simulink model "test10"  (R2024a)
settings: Solver=FixedStepAuto  StartTime=0.0  StopTime=30  FixedStep=0.001  MaxStep=1e-2  RelTol=1e-3
libraries: fl_lib x21, nesl_utility x14, simulink x7, sdl_lib x6
settings Model: DataDictionary=test4.sldd  Creator=18311  LastModifiedBy=18311

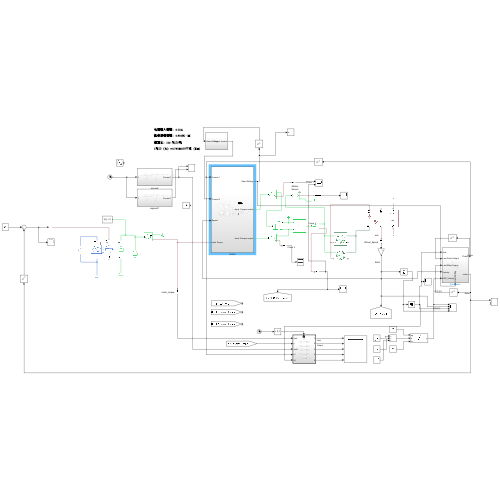
[thumbnail: Simulink's stored preview of the top-level diagram]
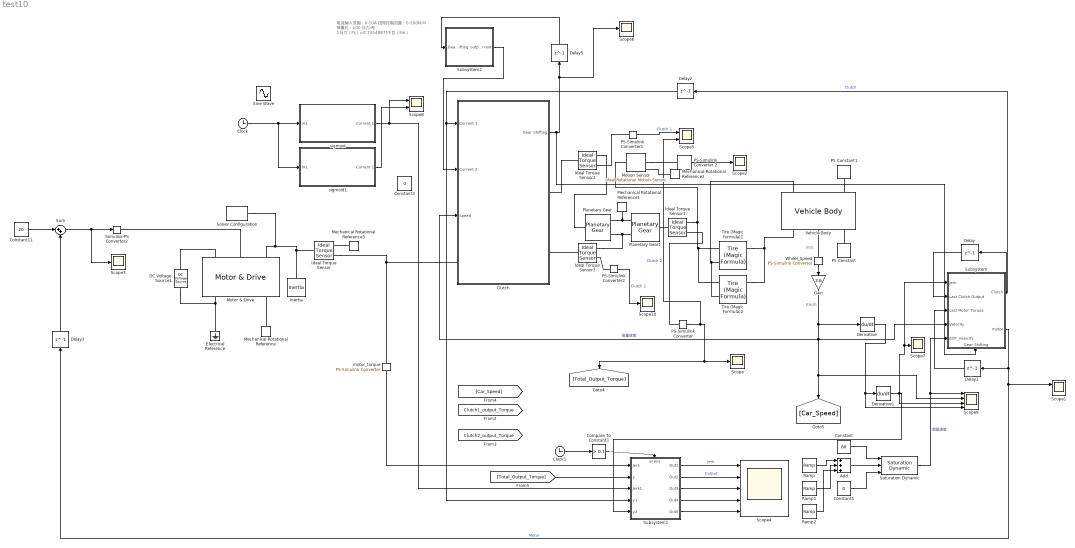
== system test10 ==
  note: Km/h
  note: m/s
  note: 电流输入范围：0-10A
      | 扭矩控制范围：0-500N·M
      | 推重比：100 马力/吨
      | 1马力（Ps）=0.73549875千瓦（Kw）
  Add : Sum  Inputs=+++
  Clock : Clock
  Clock1 : Clock
  Clutch : Subsystem
  Compare To Constant1 : simulink/Logic and Bit Operations/Compare To Constant  relop=>  const=0.1  OutDataTypeStr=boolean
  Constant : Constant  Value=80
  Constant1 : Constant  Value=0
  Constant11 : Constant  Value=20
  Constant3 : Constant  Value=0
  DC Voltage Source1 : fl_lib/Electrical/Electrical Sources/DC Voltage Source  v0=220 V
  Delay{,1..3,5} (5 alike) : Delay  DelayLength=1  InitialCondition=0
  Derivative : Derivative
  Derivative1 : Derivative
  Electrical Reference : fl_lib/Electrical/Electrical Elements/Electrical Reference
  Gain : Gain  Gain=3.6
  Ideal Torque Sensor{,1..3} (4 alike) : fl_lib/Mechanical/Mechanical Sensors/Ideal Torque Sensor
  Inertia : fl_lib/Mechanical/Rotational Elements/Inertia  inertia=0.01 kg*m^2  num_ports=foundation.enum.numPorts2.one  w_specify=off  w_priority=High  w=0 rad/s  w_nominal_specify=off  w_nominal_value=1  w_nominal_unit=rad/s  t_specify=off  t_priority=None  t=0 N*m  t_nominal_specify=off  t_nominal_value=1  t_nominal_unit=N*m
  Mechanical Rotational Reference{,1..3} (4 alike) : fl_lib/Mechanical/Rotational Elements/Mechanical Rotational Reference
  Motion Sensor : fl_lib/Mechanical/Mechanical Sensors/Ideal Rotational Motion Sensor  reference=foundation.enum.MeasurementReference.difference  acceleration_port=false  velocity_port=true  position_port=true  wrap_angle=simscape.enum.onoff.off  offset=0 rad
  Motor & Drive : sdl_lib/Engines & Motors/Motor & Drive  torque_max=200 N*m  power_max=73.549875 kW  Tc=0.02 s  eff=100  w_eff=4000 rpm  T_eff=200 N*m  thermal_port=simscape.enum.thermaleffects.omit  thermal_mass=100 J/K  temperature_specify=off  temperature_priority=High  temperature=300 K  temperature_nominal_specify=off  temperature_nominal_value=1  temperature_nominal_unit=K
      settings: InternalSimscapePortConfiguration="{\"Bottom\":[],\"Left\":[{\"id\":\"Vp\",\"label\":\"+\",\"type\":\"foundation.electrical.electrical\"},{\"id\":\"Tr\",\"label\":\"Tr\",\"type\":\"input\"},{\"id\":\"R\",\"label\":\"R\",\"type\":\"foundation.mechanical.rotational.rotational\"}],\"Right\":[{\"id\":\"Vm\",\"label\":\"-\",\"type\":\"foundation.electrical.electrical\"},{\"id\":\"Omega\",\"label\":\"w\",\"type\":\"output\"},{\"id\":\"C\",\"label\":\"C\",\"type\":\"foundation.mechanical.rotational.rotational\"}],\"Top\":[]}"
  PS Constant : fl_lib/Physical Signals/Sources/PS Constant  constant=0
  PS Constant1 : fl_lib/Physical Signals/Sources/PS Constant  constant=0
  PS-Simulink Converter : nesl_utility/PS-Simulink Converter  PhysicalDomain=network_engine_domain  SubClassName=ps_output  LeftPortType=input  RightPortType=output  PseudoPeriodic=off  Frequencies=[]  VectorFormat=inherit  Unit=inherit  AffineConversion=off
  PS-Simulink Converter 2 : nesl_utility/PS-Simulink Converter  PhysicalDomain=network_engine_domain  SubClassName=ps_output  LeftPortType=input  RightPortType=output  PseudoPeriodic=off  Frequencies=[]  VectorFormat=1-D array  Unit=rpm  AffineConversion=off
  PS-Simulink Converter1 : nesl_utility/PS-Simulink Converter  PhysicalDomain=network_engine_domain  SubClassName=ps_output  LeftPortType=input  RightPortType=output  PseudoPeriodic=off  Frequencies=[]  VectorFormat=inherit  Unit=inherit  AffineConversion=off
  PS-Simulink Converter2 : nesl_utility/PS-Simulink Converter  PhysicalDomain=network_engine_domain  SubClassName=ps_output  LeftPortType=input  RightPortType=output  PseudoPeriodic=off  Frequencies=[]  VectorFormat=inherit  Unit=inherit  AffineConversion=off
  Planetary Gear : sdl_lib/Gears/Planetary Gear  rs_ratio=1.5  friction_model=sdl.enum.gear_friction.none  efficiency=[.96, .98]  temperature_TLU=[280, 300, 320] K  efficiency_sp_TLU=[.95, .9, .85]  efficiency_rp_TLU=[.95, .9, .85]  pwr_thr=[.001, .001] W  mu_visc=[0, 0] N*m*s/rad  model_inertia=simscape.enum.onoff.off  planet_inertia=0.001 kg*m^2  thermal_mass=50 J/K  T_init=300 K
  Planetary Gear1 : sdl_lib/Gears/Planetary Gear  rs_ratio=3  friction_model=sdl.enum.gear_friction.none  efficiency=[.96, .98]  temperature_TLU=[280, 300, 320] K  efficiency_sp_TLU=[.95, .9, .85]  efficiency_rp_TLU=[.95, .9, .85]  pwr_thr=[.001, .001] W  mu_visc=[0, 0] N*m*s/rad  model_inertia=simscape.enum.onoff.off  planet_inertia=0.001 kg*m^2  thermal_mass=50 J/K  T_init=300 K
  Ramp : simulink/Sources/Ramp  slope=8  start=0  InitialOutput=0
  Ramp1 : simulink/Sources/Ramp  slope=-8  start=10  InitialOutput=0
  Ramp2 : simulink/Sources/Ramp  slope=-8  start=20  InitialOutput=0
  Saturation Dynamic : simulink/Discontinuities/Saturation Dynamic  OutMin=[]  OutMax=[]  OutDataTypeStr=Inherit: Same as second input  OutDataType=fixdt(1, 16)  OutScaling=2^-10  DoSatur=off
  Scope{,2..3,6..7,10} (6 alike) : Scope
  Scope1 : Scope  NumInputPorts=2
  Scope4 : Scope  NumInputPorts=5
  Scope5 : Scope  NumInputPorts=2
  Scope8 : Scope  NumInputPorts=2
  Scope9 : Scope  NumInputPorts=4
  Simulink-PS Converter2 : nesl_utility/Simulink-PS Converter  PhysicalDomain=network_engine_domain  SubClassName=ps_input  LeftPortType=input  RightPortType=output  PseudoPeriodic=off  Frequencies=[]  NoiseDistribution=none  NoiseParameters=[]  Unit=1  AffineConversion=off  FilteringAndDerivatives=provide  SimscapeFilterOrder=1  InputFilterTimeConstant=0.001  UdotUserProvided=0
  Sine Wave : Sin  Amplitude=5  Bias=5  SampleTime=0
  Solver Configuration : nesl_utility/Solver Configuration  PhysicalDomain=network_engine_domain  SubClassName=solver  LeftPortType=input  RightPortType=generic  Tones=[]  Harmonics=[]  SimulateNoise=off  Profile=off  UseLocalSampling=off  EnableSwitchedLinearOptims=on  FrequencyDomain=off  UseCCode=off  RelTol=0.001  AbsTol=0.001  MinStep=1e-09  ToWorkspace=off  RevertToSquareIcSolve=off  NumHomotopyIterations=100  PhasorMode=off  PhasorModeNumHarmonics=1  ConsistencySolver=NEWTON_XTOL_AFTER_FTOL  IndexReductionMethod=DerivativeReplacement  DoDC=off  ResidualTolerance=1e-09  ConsistencyTolSource=GLOBAL  ConsistencyAbsTol=0.001  ConsistencyRelTol=0.001  ConsistencyTolFactor=0.001  UseLocalSolver=off  LocalSolverChoice=NE_BACKWARD_EULER_ADVANCER  ResolveIndetEquations=on  FunctionEvalNumThread=1  LocalSolverSampleTime=0.001  DoFixedCost=off  MaxNonlinIter=3  MaxModeIter=2  ComputeImpulses=off  ImpulseIterations=2  LinearAlgebra=auto  LinearAlgebraNumThread=0  EquationFormulation=NE_TIME_EF  DelaysMemoryBudget=1024  AutomaticFiltering=on  FilteringTimeConstant=0.001  PartitionStorageMethod=AS_NEEDED  PartitionMemoryBudget=1024  PartitionMethod=ROBUST  MultibodyUseLocalSolver=off  MultibodyLocalSolverChoice=ODE1  MultibodyLocalSolverSampleTime=0.001
  Subsystem : Subsystem
      settings: PortSchema="{\"entries\":[{\"content\":{\"sides\":[{\"content\":{\"connectorIds\":[\"In1\",\"In2\",\"In3\",\"In4\",\"In5\"]},\"type\":\"ConnectorPlacement.EquallySpacedRectSide\",\"uuid\":\"5fc21831-6841-4d26-9c3b-273312b90933\"},{\"content\":{\"connectorIds\":[\"Out1\",\"Out2\"],\"side\":\"RIGHT\"},\"type\":\"ConnectorPlacement.EquallySpacedRectSide\",\"uuid\":\"d2976722-6716-4e73-9e66-a79e5a3f513c\"},{\"content\":{\"side\":\"TOP\"},\"type\":\"ConnectorPlacement.EquallySpacedRectSide\",\"uuid\":\"ab612606-baef-4711-bd49-fbf1df8d6358\"},{\"content\":{\"connectorIds\":[\"In6\"],\"side\":\"BOTTOM\"},\"type\":\"ConnectorPlacement.EquallySpacedRectSide\",\"uuid\":\"7be4a3f2-b973-419e-bcc3-9bfae442f3d1\"}]},\"type\":\"ConnectorPlacement.EquallySpacedConnector\",\"uuid\":\"4db5bfe9-dab6-4d88-a0f8-710cccb4717b\"}],\"packageUris\":[\"http://schema.mathworks.com/mf0/Connector/R2020b\"],\"version\":\"1.0\"}"
  Subsystem1 : Subsystem
  Subsystem2 : Subsystem
  Sum : Sum  Inputs=|++
  Tire (Magic Formula)1 : sdl_lib/Tires & Vehicles/Tire (Magic Formula)  parameterization=sdl.enum.magic_tire_model.peak  F_z1=2500 N  F_x1=3500 N  kappa1=10  B_m=10  C_m=1.9  D_m=1  E_m=0.97  fz0=4000 N  p_Cx=1.685  p_Dx=[1.21, -.037]  p_Ex=[.344, .095, -.02, 0]  p_Kx=[21.51, -.163, .245]  p_Hx=[-.002, .002]  p_Vx=[0, 0]  rolling_radius_model=sdl.enum.RollingRadiusParameterization.Constant  r_e=0.3 m  r_0=0.3 m  breff=8.39  dreff=0.26  freff=0.074  q_re0=0.99  q_v1=0.008  longvl=17 m/s  cz=5e5 N/m  model_resistance=true  resistance_model=sdl.enum.rollingResistanceParameterization.constant  coeff=0.015  p_tire=250e3 Pa  alpha=-0.003  beta=0.97  coeff_a=84e-4  coeff_b=6.2e-4 s/m  coeff_c=1.6e-4 s^2/m^2  p_tire0=240e3 Pa  fz0_resistance=4000 N  vH0=16 m/s  q_Sy=[.0082, 0, .0014, .001, 0, 0, 1.08, -.5]  v_thr=0.001 m/s  enable_scaling_coefficients=false  lfzO=1  lcx=1  lmux=1  lex=1  lkx=1  lhx=1  lvx=1  lmy=1  model_compliance=sdl.enum.compliance.off  stiffness=1e6 N/m  damping=1000 N*s/m  model_inertia=sdl.enum.model_inertia.off  inertia=1 kg*m^2  initial_velocity=0 rad/s  vxlow=1 m/s  v_tr_thr=0.1 m/s  kpumin=-1.5  kpumax=1.5
  Tire (Magic Formula)2 : sdl_lib/Tires & Vehicles/Tire (Magic Formula)  parameterization=sdl.enum.magic_tire_model.peak  F_z1=2500 N  F_x1=3000 N  kappa1=10  B_m=10  C_m=1.9  D_m=1  E_m=0.97  fz0=4000 N  p_Cx=1.685  p_Dx=[1.21, -.037]  p_Ex=[.344, .095, -.02, 0]  p_Kx=[21.51, -.163, .245]  p_Hx=[-.002, .002]  p_Vx=[0, 0]  rolling_radius_model=sdl.enum.RollingRadiusParameterization.Constant  r_e=0.3 m  r_0=0.3 m  breff=8.39  dreff=0.26  freff=0.074  q_re0=0.99  q_v1=0.008  longvl=17 m/s  cz=5e5 N/m  model_resistance=true  resistance_model=sdl.enum.rollingResistanceParameterization.constant  coeff=0.015  p_tire=250e3 Pa  alpha=-0.003  beta=0.97  coeff_a=84e-4  coeff_b=6.2e-4 s/m  coeff_c=1.6e-4 s^2/m^2  p_tire0=240e3 Pa  fz0_resistance=4000 N  vH0=16 m/s  q_Sy=[.0082, 0, .0014, .001, 0, 0, 1.08, -.5]  v_thr=0.001 m/s  enable_scaling_coefficients=false  lfzO=1  lcx=1  lmux=1  lex=1  lkx=1  lhx=1  lvx=1  lmy=1  model_compliance=sdl.enum.compliance.off  stiffness=1e6 N/m  damping=1000 N*s/m  model_inertia=sdl.enum.model_inertia.off  inertia=1 kg*m^2  initial_velocity=0 rad/s  vxlow=1 m/s  v_tr_thr=0.1 m/s  kpumin=-1.5  kpumax=1.5
  Vehicle Body : sdl_lib/Tires & Vehicles/Vehicle Body  mass=1000 kg  n_w=1  x_f=1.4 m  x_r=1.6 m  y_c=0.5 m  mass_var=simscape.enum.onoff.off  g=9.81 m/s^2  liftoff_warning=simscape.enum.onoff.off  area=3 m^2  Cd=0.4  rho=1.18 kg/m^3  model_pitch=simscape.enum.onoff.off  inertia=4000 kg*m^2  suspension_model=sdl.enum.linearTLU.linear  k_f=1e4 N/m  b_f=1e4 N*s/m  k_r=1e4 N/m  b_r=1e4 N*s/m  k_f_TLU=[-2000, -1000, 0, 1000, 2000] N  x_f_TLU=[-.4, -.2, 0, .2, .4] m  b_f_TLU=[-200, -100, 0, 100, 200] N  v_f_TLU=[-4, -2, 0, 2, 4] m/s  k_r_TLU=[-2000, -1000, 0, 1000, 2000] N  x_r_TLU=[-.4, -.2, 0, .2, .4] m  b_r_TLU=[-200, -100, 0, 100, 200] N  v_r_TLU=[-4, -2, 0, 2, 4] m/s  interp_method=simscape.enum.interpolation.linear  extrap_method=simscape.enum.extrapolation.linear  model_hardstop=simscape.enum.onoff.off  upper_bound_f=.25 m  lower_bound_f=-.25 m  stop_k_f=1e6 N/m  stop_b_f=150 N*s/m  upper_bound_r=.25 m  lower_bound_r=-.25 m  stop_k_r=1e6 N/m  stop_b_r=150 N*s/m  initial_pitch=0 rad  initial_pitch_rate=0 rad/s  v_specify=off  v_priority=High  v=0 m/s  v_nominal_specify=off  v_nominal_value=1  v_nominal_unit=m/s
  Wheel_Speed : nesl_utility/PS-Simulink Converter  PhysicalDomain=network_engine_domain  SubClassName=ps_output  LeftPortType=input  RightPortType=output  PseudoPeriodic=off  Frequencies=[]  VectorFormat=inherit  Unit=inherit  AffineConversion=off
  motor_torque : nesl_utility/PS-Simulink Converter  PhysicalDomain=network_engine_domain  SubClassName=ps_output  LeftPortType=input  RightPortType=output  PseudoPeriodic=off  Frequencies=[]  VectorFormat=inherit  Unit=inherit  AffineConversion=off
  sigmoid : Subsystem
  sigmoid1 : Subsystem
  wires:
  motor_torque/1 -> Subsystem1/1(Jerk)
  Wheel_Speed/1 -> Gain/1
  [Total_Output_Torque] -> Subsystem1/2(y)
  Derivative/1 -> Scope9/4, Derivative1/1
  Constant11/1 -> Sum/1
  Sum/1 -> Scope3/1, Simulink-PS Converter2/1
  Subsystem/2(motor) -> Delay3/1, Scope1/1, Delay1/1  "Motor"
  Subsystem/1(Clutch) -> Delay2/1, Delay/1  "Clutch"
  Derivative1/1 -> Scope7/1, Subsystem/1(Jerk), Scope9/3, Subsystem1/5(y2)
  sigmoid/1(Current 1) -> Scope8/1, Subsystem1/3(Jerk1)
  Clock/1 -> sigmoid1/1(In1), sigmoid/1(In1)
  Saturation Dynamic/1 -> Subsystem/5(EXP_Velocity), Scope9/1  "期望速度"
  Delay/1 -> Subsystem/2(Last Clutch Output)
  Delay1/1 -> Subsystem/3(Last Motor Torque)
  Delay2/1 -> Clutch/1(Current 1), Subsystem1/4(y1)
  Clock1/1 -> Compare To Constant1/1
  Compare To Constant1/1 -> Subsystem1/Enable
  Subsystem1/1(Out1) -> Scope4/1  "Jerk"
  Subsystem1/2(Out2) -> Scope4/2  "Output"
  Subsystem1/3(Out3) -> Scope4/3
  Subsystem1/4(Out4) -> Scope4/4
  Subsystem1/5(Out5) -> Scope4/5
  Constant/1 -> Saturation Dynamic/1
  Constant1/1 -> Saturation Dynamic/3
  Gain/1 -> Scope9/2, [Car_Speed], Clutch/3(Speed), Subsystem/4(Velocity), Derivative/1  "测量速度"
  sigmoid1/1(Current 1) -> Scope8/2
  Delay3/1 -> Sum/2
  PS-Simulink Converter/1 -> Scope5/2, [Total_Output_Torque], Scope/1  "Clutch 2"
  PS-Simulink Converter 2/1 -> Scope2/1
  PS-Simulink Converter1/1 -> Scope5/1  "Clutch 1"
  Clutch/1(Gear Shifting) -> Subsystem/6(Gear Shifting), Scope6/1, Delay5/1
  Delay5/1 -> Subsystem2/1(Gear shifting)
  Subsystem2/1(output current) -> Clutch/2(Current 2)
  PS-Simulink Converter2/1 -> Scope10/1  "Clutch 2"
  Ramp/1 -> Add/1
  Ramp1/1 -> Add/2
  Ramp2/1 -> Add/3
  Add/1 -> Saturation Dynamic/2
  connections:
  Motor & Drive/LConn1 -- DC Voltage Source1/LConn1
  Electrical Reference/LConn1 -- DC Voltage Source1/RConn1 -- Motor & Drive/RConn1
  Mechanical Rotational Reference/LConn1 -- Motor & Drive/RConn3
  Inertia/LConn1 -- Motor & Drive/LConn3 -- Solver Configuration/RConn1 -- Ideal Torque Sensor/LConn1
  PS Constant/RConn1 -- Vehicle Body/LConn3
  PS Constant1/RConn1 -- Vehicle Body/RConn3
  Ideal Torque Sensor/RConn2 -- motor_torque/LConn1 -- Clutch/LConn1
  Wheel_Speed/LConn1 -- Vehicle Body/LConn2
  Simulink-PS Converter2/RConn1 -- Motor & Drive/LConn2
  Tire (Magic Formula)1/RConn2 -- Tire (Magic Formula)2/RConn2 -- Vehicle Body/LConn1
  Tire (Magic Formula)1/LConn1 -- Tire (Magic Formula)2/LConn1 -- Vehicle Body/RConn1
  Mechanical Rotational Reference3/LConn1 -- Ideal Torque Sensor/RConn1
  Planetary Gear/RConn1 -- Mechanical Rotational Reference1/LConn1 -- Planetary Gear1/RConn1
  Ideal Torque Sensor1/LConn1 -- Planetary Gear1/LConn1
  PS-Simulink Converter/LConn1 -- Ideal Torque Sensor1/RConn2
  Planetary Gear/RConn2 -- Ideal Torque Sensor3/RConn1 -- Planetary Gear1/RConn2
  Motion Sensor/RConn2 -- PS-Simulink Converter 2/LConn1
  Ideal Torque Sensor1/RConn1 -- Tire (Magic Formula)2/LConn2 -- Tire (Magic Formula)1/LConn2 -- Motion Sensor/LConn1
  Mechanical Rotational Reference2/LConn1 -- Motion Sensor/RConn1
  Ideal Torque Sensor2/RConn1 -- Planetary Gear/LConn1
  PS-Simulink Converter1/LConn1 -- Ideal Torque Sensor2/RConn2
  Ideal Torque Sensor2/LConn1 -- Clutch/RConn1
  Ideal Torque Sensor3/LConn1 -- Clutch/RConn2
  PS-Simulink Converter2/LConn1 -- Ideal Torque Sensor3/RConn2

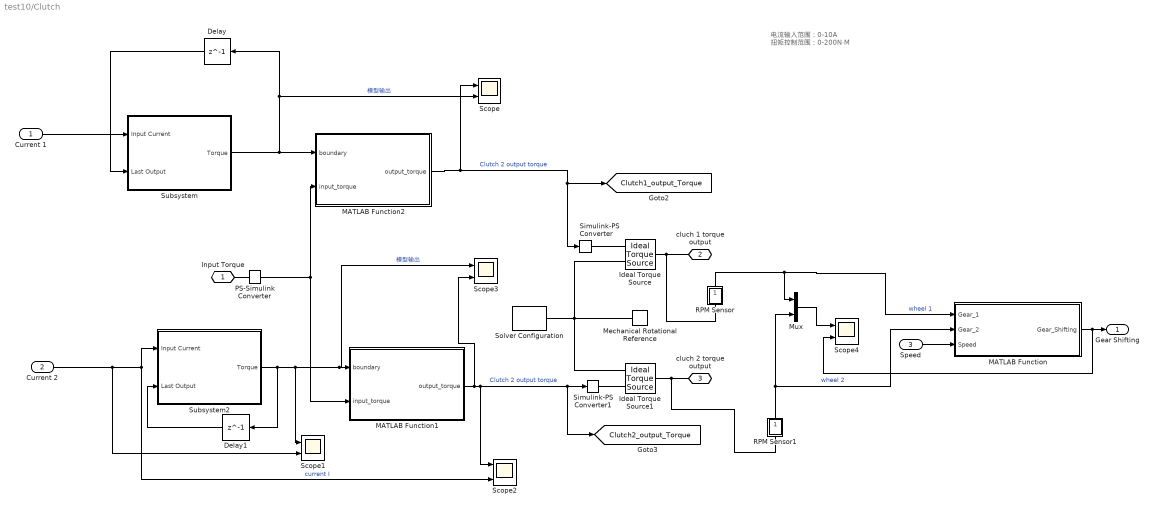
== system test10/Clutch ==
  note: 电流输入范围：0-10A
      | 扭矩控制范围：0-200N·M
  Current 1 : Inport
  Current 2 : Inport  Port=2
  Speed : Inport  Port=3
  Delay : Delay  DelayLength=1  InitialCondition=0
  Delay1 : Delay  DelayLength=1  InitialCondition=0
  Ideal Torque Source : fl_lib/Mechanical/Mechanical Sources/Ideal Torque Source
  Ideal Torque Source1 : fl_lib/Mechanical/Mechanical Sources/Ideal Torque Source
  MATLAB Function : MATLAB Function  TreatAsAtomicUnit=on
  MATLAB Function1 : MATLAB Function  TreatAsAtomicUnit=on
  MATLAB Function2 : MATLAB Function  TreatAsAtomicUnit=on
  Mechanical Rotational Reference : fl_lib/Mechanical/Rotational Elements/Mechanical Rotational Reference
  Mux : Mux  Inputs=2
  PS-Simulink Converter : nesl_utility/PS-Simulink Converter  PhysicalDomain=network_engine_domain  SubClassName=ps_output  LeftPortType=input  RightPortType=output  PseudoPeriodic=off  Frequencies=[]  VectorFormat=inherit  Unit=inherit  AffineConversion=off
  RPM Sensor : Subsystem
      mask Display: disp('S')
  RPM Sensor1 : Subsystem
      mask Display: disp('S')
  Scope{,1,3..4} (4 alike) : Scope  NumInputPorts=2
  Scope2 : Scope  NumInputPorts=3
  Simulink-PS Converter : nesl_utility/Simulink-PS Converter  PhysicalDomain=network_engine_domain  SubClassName=ps_input  LeftPortType=input  RightPortType=output  PseudoPeriodic=off  Frequencies=[]  NoiseDistribution=none  NoiseParameters=[]  Unit=1  AffineConversion=off  FilteringAndDerivatives=provide  SimscapeFilterOrder=1  InputFilterTimeConstant=0.001  UdotUserProvided=0
  Simulink-PS Converter1 : nesl_utility/Simulink-PS Converter  PhysicalDomain=network_engine_domain  SubClassName=ps_input  LeftPortType=input  RightPortType=output  PseudoPeriodic=off  Frequencies=[]  NoiseDistribution=none  NoiseParameters=[]  Unit=1  AffineConversion=off  FilteringAndDerivatives=provide  SimscapeFilterOrder=1  InputFilterTimeConstant=0.001  UdotUserProvided=0
  Solver Configuration : nesl_utility/Solver Configuration  PhysicalDomain=network_engine_domain  SubClassName=solver  LeftPortType=input  RightPortType=generic  Tones=[]  Harmonics=[]  SimulateNoise=off  Profile=off  UseLocalSampling=off  EnableSwitchedLinearOptims=on  FrequencyDomain=off  UseCCode=off  RelTol=0.001  AbsTol=0.001  MinStep=1e-09  ToWorkspace=off  RevertToSquareIcSolve=off  NumHomotopyIterations=100  PhasorMode=off  PhasorModeNumHarmonics=1  ConsistencySolver=NEWTON_XTOL_AFTER_FTOL  IndexReductionMethod=DerivativeReplacement  DoDC=off  ResidualTolerance=1e-09  ConsistencyTolSource=GLOBAL  ConsistencyAbsTol=0.001  ConsistencyRelTol=0.001  ConsistencyTolFactor=0.001  UseLocalSolver=off  LocalSolverChoice=NE_BACKWARD_EULER_ADVANCER  ResolveIndetEquations=on  FunctionEvalNumThread=1  LocalSolverSampleTime=0.001  DoFixedCost=off  MaxNonlinIter=3  MaxModeIter=2  ComputeImpulses=off  ImpulseIterations=2  LinearAlgebra=auto  LinearAlgebraNumThread=0  EquationFormulation=NE_TIME_EF  DelaysMemoryBudget=1024  AutomaticFiltering=on  FilteringTimeConstant=0.001  PartitionStorageMethod=AS_NEEDED  PartitionMemoryBudget=1024  PartitionMethod=ROBUST  MultibodyUseLocalSolver=off  MultibodyLocalSolverChoice=ODE1  MultibodyLocalSolverSampleTime=0.001
  Subsystem : Subsystem  mask{c=-2, k=20, d=0.6, alpha=-37.209}
  Subsystem2 : Subsystem  mask{c=-2, k=20, d=0.6, alpha=-37.209}
  Input Torque : PMIOPort  Side=Left
  cluch 1 torque output : PMIOPort  Port=2  Side=Right
  cluch 2 torque output : PMIOPort  Port=3  Side=Right
  Gear Shifting : Outport
  tag scope: Clutch1_output_Torque=global, Clutch2_output_Torque=global
  wires:
  Current 1/1 -> Subsystem/1(Input Current)
  Current 2/1 -> Scope1/2, Scope2/3, Subsystem2/1(Input Current)  "current I"
  MATLAB Function1/1(output_torque) -> Scope3/2, [Clutch2_output_Torque], Simulink-PS Converter1/1, Scope2/1  "Clutch 2 output torque"
  MATLAB Function2/1(output_torque) -> Scope/1, Simulink-PS Converter/1, [Clutch1_output_Torque]  "Clutch 2 output torque"
  PS-Simulink Converter/1 -> MATLAB Function2/2(input_torque), MATLAB Function1/2(input_torque)
  RPM Sensor/1(rpm) -> Mux/1, MATLAB Function/1(Gear_1)  "wheel 1"
  Subsystem2/1(Torque) -> Delay1/1, Scope1/1, Scope3/1, MATLAB Function1/1(boundary)  "模型输出"
  RPM Sensor1/1(rpm) -> Mux/2, MATLAB Function/2(Gear_2)  "wheel 2"
  Subsystem/1(Torque) -> Delay/1, Scope/2, MATLAB Function2/1(boundary)  "模型输出"
  Speed/1 -> MATLAB Function/3(Speed)
  MATLAB Function/1(Gear_Shifting) -> Scope4/2, Gear Shifting/1
  Mux/1 -> Scope4/1
  Delay/1 -> Subsystem/2(Last Output)
  Delay1/1 -> Subsystem2/2(Last Output)
  connections:
  Input Torque/RConn1 -- PS-Simulink Converter/LConn1
  Ideal Torque Source/RConn2 -- Ideal Torque Source1/RConn2 -- Mechanical Rotational Reference/LConn1 -- Solver Configuration/RConn1
  Ideal Torque Source/LConn1 -- RPM Sensor/LConn1 -- cluch 1 torque output/RConn1
  Ideal Torque Source1/LConn1 -- RPM Sensor1/LConn1 -- cluch 2 torque output/RConn1
  Ideal Torque Source/RConn1 -- Simulink-PS Converter/RConn1
  Ideal Torque Source1/RConn1 -- Simulink-PS Converter1/RConn1

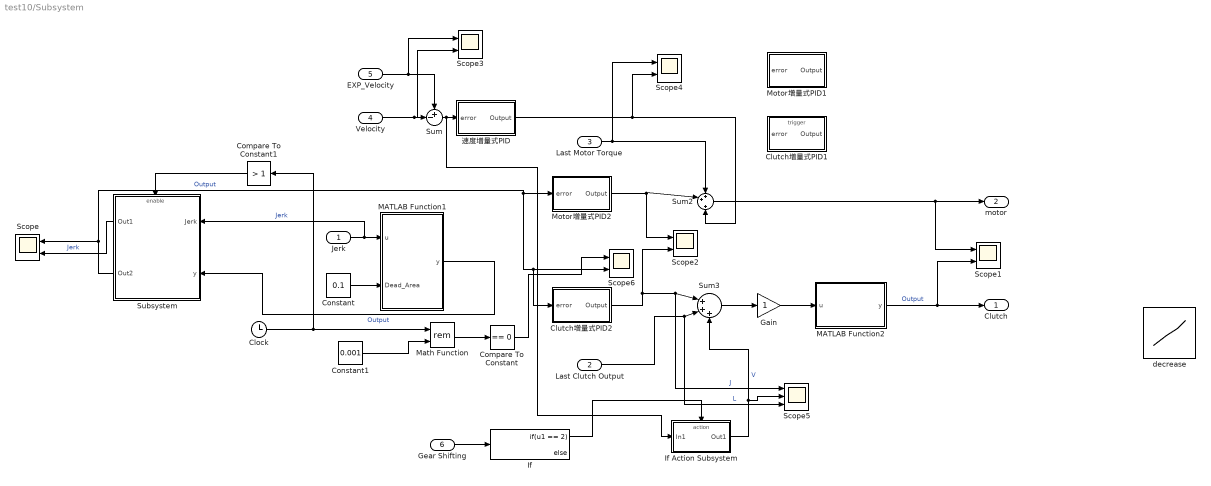
== system test10/Subsystem ==
  Jerk : Inport
  Last Clutch Output : Inport  Port=2
  Last Motor Torque : Inport  Port=3
  Velocity : Inport  Port=4
  EXP_Velocity : Inport  Port=5
  Gear Shifting : Inport  Port=6
  Clock : Clock
  Clutch增量式PID1 : Subsystem  mask{Kp=0.09, Ki=0.02, Kd=0.03}
      mask DialogControl ParameterGroupVar Prompt: 参数
  Clutch增量式PID2 : Subsystem  mask{Kp=0.0002, Ki=0, Kd=0.00001}
      mask DialogControl ParameterGroupVar Prompt: 参数
  Compare To Constant : simulink/Logic and Bit Operations/Compare To Constant  relop===  const=0  OutDataTypeStr=boolean
  Compare To Constant1 : simulink/Logic and Bit Operations/Compare To Constant  relop=>  const=1  OutDataTypeStr=boolean
  Constant : Constant  Value=0.1
  Constant1 : Constant  Value=0.001
  Gain : Gain
  If : If  IfExpression=u1 == 2
  If Action Subsystem : Subsystem  TreatAsAtomicUnit=on
  MATLAB Function1 : MATLAB Function  TreatAsAtomicUnit=on
  MATLAB Function2 : MATLAB Function  TreatAsAtomicUnit=on
  Math Function : Math  Operator=rem
  Motor增量式PID1 : Subsystem  mask{Kp=5, Ki=1, Kd=3}
      mask DialogControl ParameterGroupVar Prompt: 参数
  Motor增量式PID2 : Subsystem  mask{Kp=0, Ki=0, Kd=0}
      mask DialogControl ParameterGroupVar Prompt: 参数
  Scope{,1..4,6} (6 alike) : Scope  NumInputPorts=2
  Scope5 : Scope  NumInputPorts=3
  Subsystem : Subsystem
  Sum : Sum  Inputs=+-|
  Sum2 : Sum  Inputs=++|+
  Sum3 : Sum  Inputs=|+++
  decrease : Lookup_n-D  NumberOfTableDimensions=1  BreakpointsForDimension1=[5.5594823336345e-05;6.14417460221472e-05;6.79035869809514e-05;7.50450159711001e-05;8.29375037389161e-05;9.16600371985333e-05;0.000101299909808739;0.000111953595051133;0.000123727711744276;0.000136740090845997;0.000151120954409751;0.000167014218480952;0.00018457893295667;0.000203990872799214;0.000225444296504455;0.000249153889394299;0.000275356911145835;0.000304315569005653;0.000336319640386712;0.000371689371028895;0.000410778677647633;0.000453978687024344;0.000501721646837642;0.000554485247227949;0.000612797396166024;0.000677241496197702;0.000748462275106112;0.000827172228516664;0.000914158738521614;0.00101029193907773;0.00111653340629563;0.00123394575986232;0.00136370327079497;0.00150710358059758;0.00166558064777336;0.00184071904963424;0.00203426978055207;0.00224816770233296;0.00248455081839335;0.00274578156101333;0.00303447030028919;0.00335350130466478;0.00370606140626397;0.00409567164986051;0.00452622223240535;0.00500201107079564;0.00552778636923599;0.00610879359434402;0.00675082730632838;0.00746028833836698;0.00824424686398295;0.00911051194400646;0.0100677082008564;0.0111253603286032;0.0122939862127742;0.0135851995042896;0.0150118225673699;0.0165880108017442;0.0183293894249281;0.0202532038904988;0.0223784852127633;0.0247262315663477;0.0273196076301106;0.0301841632470842;0.0333480730741335;0.0368423989943599;0.0407013771589613;0.0449627316094118;0.0496680165005697;0.0548629889945041;0.0605980149158412;0.0669285092428486;0.0739154134428198;0.081625711531599;0.0901329865284782;0.0995180186690433;0.109869426305932;0.121284349842742;0.133869178276648;0.147740316932731;0.163024993714409;0.179862099620916;0.198403057340775;0.218812709361305;0.241270214176692;0.265969935768659;0.293122307513563;0.322954646984505;0.355711892726362;0.391657227967644;0.431072549410861;0.474258731775668;0.521535630784177;0.573241758988688;0.629733560569965;0.691384203433468;0.758581800212436;0.831726964939224;0.911229610148562;0.997504891196852;1.09096821195613;1.19202922022118;1.30108474362998;1.41851064900488;1.54465265083535;1.67981614866076;1.82425523806356;1.97816111441418;2.14165016957441;2.31475216500982;2.49739894404882;2.68941421369995;2.89050497374996;3.10025518872388;3.31812227831834;3.54343693774205;3.77540668798146;4.01312339887548;4.25557483188341;4.50166002687522;4.7502081252106;5;5.2497918747894;5.49833997312478;5.74442516811659;5.98687660112452;6.22459331201854;6.45656306225795;6.68187772168166;6.89974481127612;7.10949502625004;7.31058578630005;7.50260105595118;7.68524783499018;7.85834983042559;8.02183888558582;8.17574476193644;8.32018385133924;8.45534734916465;8.58148935099512;8.69891525637002;8.80797077977882;8.90903178804387;9.00249510880315;9.08877038985144;9.16827303506078;9.24141819978757;9.30861579656653;9.37026643943003;9.42675824101131;9.47846436921582;9.52574126822433;9.56892745058914;9.60834277203236;9.64428810727364;9.67704535301549;9.70687769248644;9.73403006423134;9.75872978582331;9.78118729063869;9.80159694265923;9.82013790037908;9.83697500628559;9.85225968306727;9.86613082172335;9.87871565015726;9.89013057369407;9.90048198133096;9.90986701347152;9.9183742884684;9.92608458655718;9.93940198508416;9.94513701100549;9.95503726839059;9.96665192692587;9.97527376843365;9.9949979889292;9.99993209641302]  Table=[0;6.14417460221472e-05;6.79035869809514e-05;7.50450159711001e-05;8.29375037389161e-05;9.16600371985333e-05;0.000101299909808739;0.000111953595051133;0.000123727711744276;0.000136740090845997;0.000151120954409752;0.000167014218480952;0.00018457893295667;0.000203990872799214;0.000225444296504455;0.000249153889394299;0.000275356911145835;0.000304315569005653;0.000336319640386712;0.000371689371028895;0.000410778677647633;0.000453978687024344;0.000501721646837643;0.000554485247227949;0.000612797396166024;0.000677241496197702;0.000748462275106112;0.000827172228516664;0.000914158738521614;0.00101029193907773;0.00111653340629563;0.00123394575986232;0.00136370327079497;0.00150710358059758;0.00166558064777336;0.00184071904963424;0.00203426978055207;0.00224816770233296;0.00248455081839335;0.00274578156101333;0.00303447030028919;0.00335350130466478;0.00370606140626397;0.00409567164986051;0.00452622223240536;0.00500201107079564;0.00552778636923599;0.00610879359434402;0.00675082730632838;0.00746028833836698;0.00824424686398295;0.00911051194400646;0.0100677082008564;0.0111253603286032;0.0122939862127742;0.0135851995042896;0.0150118225673699;0.0165880108017442;0.0183293894249281;0.0202532038904988;0.0223784852127634;0.0247262315663477;0.0273196076301106;0.0301841632470842;0.0333480730741335;0.0368423989943599;0.0407013771589613;0.0449627316094118;0.0496680165005697;0.0548629889945041;0.0605980149158412;0.0669285092428486;0.0739154134428198;0.081625711531599;0.0901329865284782;0.0995180186690433;0.109869426305932;0.121284349842742;0.133869178276648;0.147740316932731;0.163024993714409;0.179862099620916;0.198403057340775;0.218812709361305;0.241270214176692;0.265969935768659;0.293122307513563;0.322954646984505;0.355711892726362;0.391657227967644;0.431072549410861;0.474258731775668;0.521535630784177;0.573241758988688;0.629733560569965;0.691384203433468;0.758581800212436;0.831726964939224;0.911229610148562;0.997504891196852;1.09096821195613;1.19202922022118;1.30108474362998;1.41851064900488;1.54465265083535;1.67981614866076;1.82425523806356;1.97816111441418;2.14165016957441;2.31475216500982;2.49739894404882;2.68941421369995;2.89050497374996;3.10025518872388;3.31812227831834;3.54343693774205;3.77540668798146;4.01312339887548;4.25557483188341;4.50166002687522;4.7502081252106;5;5.2497918747894;5.49833997312478;5.74442516811659;5.98687660112452;6.22459331201854;6.45656306225795;6.68187772168166;6.89974481127612;7.10949502625004;7.31058578630005;7.50260105595118;7.68524783499018;7.85834983042559;8.02183888558582;8.17574476193644;8.32018385133924;8.45534734916465;8.58148935099512;8.69891525637002;8.80797077977882;8.90903178804387;9.00249510880315;9.08877038985144;9.16827303506078;9.24141819978757;9.30861579656653;9.37026643943003;9.42675824101131;9.47846436921582;9.52574126822433;9.56892745058914;9.60834277203236;9.64428810727364;9.67704535301549;9.70687769248644;9.73403006423134;9.75872978582331;9.78118729063869;9.80159694265923;9.82013790037908;9.83697500628559;9.85225968306727;9.86613082172335;9.87871565015726;9.89013057369407;9.90048198133096;9.90986701347152;9.9183742884684;9.92608458655718;9.93307149075715;9.93940198508416;9.94513701100549;9.95503726839059;9.96665192692587;9.97527376843365;9.98641480049571;]  InternalRulePriority=Speed  RndMeth=Simplest
  速度增量式PID : Subsystem  mask{Kp=20, Ki=0.2, Kd=0}
      mask DialogControl ParameterGroupVar Prompt: 参数
  Clutch : Outport
  motor : Outport  Port=2
  wires:
  Velocity/1 -> Scope3/2, Sum/2
  EXP_Velocity/1 -> Scope3/1, Sum/1
  Jerk/1 -> Subsystem/1(Jerk), MATLAB Function1/1(u)  "Jerk"
  速度增量式PID/1(Output) -> Scope4/2, Sum2/3
  Last Motor Torque/1 -> Sum2/1, Scope4/1
  Motor增量式PID2/1(Output) -> Scope2/1, Sum2/2
  Last Clutch Output/1 -> Scope5/3, Sum3/2  "L"
  Sum/1 -> If Action Subsystem/1(In1), 速度增量式PID/1(error)
  MATLAB Function1/1(y) -> Subsystem/2(y)  "Output"
  Constant/1 -> MATLAB Function1/2(Dead_Area)
  Sum2/1 -> Scope1/1, motor/1
  Sum3/1 -> Gain/1
  Clock/1 -> Compare To Constant1/1, Math Function/1
  Constant1/1 -> Math Function/2
  Math Function/1 -> Compare To Constant/1
  Compare To Constant/1 -> Scope6/1
  Gain/1 -> MATLAB Function2/1(u)
  MATLAB Function2/1(y) -> Scope1/2, Clutch/1  "Output"
  Compare To Constant1/1 -> Subsystem/Enable
  Subsystem/2(Out2) -> Scope/1, Clutch增量式PID2/1(error), Scope6/2, Motor增量式PID2/1(error)  "Output"
  Clutch增量式PID2/1(Output) -> Scope2/2, Scope5/1, Sum3/1  "J"
  Gear Shifting/1 -> If/1
  If/1 -> If Action Subsystem/Action
  If Action Subsystem/1(Out1) -> Scope5/2, Sum3/3  "V"
  Subsystem/1(Out1) -> Scope/2  "Jerk"

== system test10/Subsystem1 ==
  Jerk : Inport
  y : Inport  Port=2
  Jerk1 : Inport  Port=3
  y1 : Inport  Port=4
  y2 : Inport  Port=5
  Enable : EnablePort
  Out1 : Outport
  Out2 : Outport  Port=2
  Out3 : Outport  Port=3
  Out4 : Outport  Port=4
  Out5 : Outport  Port=5
  wires:
  Jerk/1 -> Out1/1
  y/1 -> Out2/1
  Jerk1/1 -> Out3/1
  y1/1 -> Out4/1
  y2/1 -> Out5/1

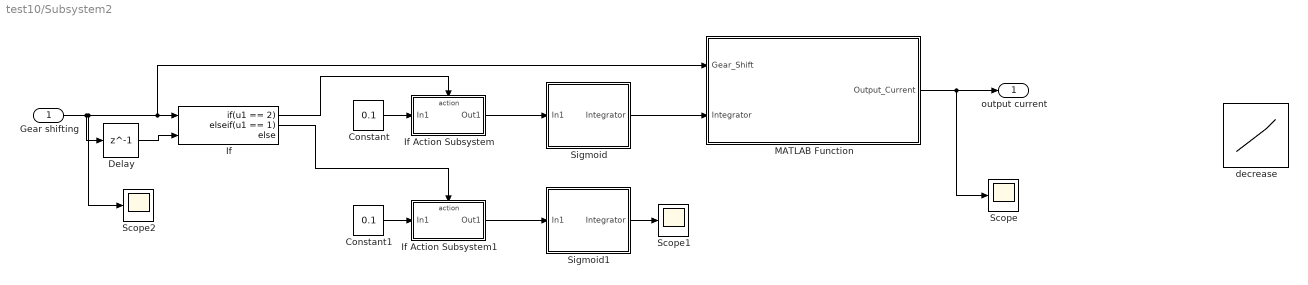
== system test10/Subsystem2 ==
  Gear shifting : Inport
  Constant : Constant  Value=0.1
  Constant1 : Constant  Value=0.1
  Delay : Delay  DelayLength=1  InitialCondition=0
  If : If  NumInputs=2  IfExpression=u1 == 2  ElseIfExpressions=u1 == 1
  If Action Subsystem : Subsystem  TreatAsAtomicUnit=on
  If Action Subsystem1 : Subsystem  TreatAsAtomicUnit=on
  MATLAB Function : MATLAB Function  TreatAsAtomicUnit=on
  Scope : Scope
  Scope1 : Scope
  Scope2 : Scope
  Sigmoid : Subsystem
  Sigmoid1 : Subsystem
  decrease : Lookup_n-D  NumberOfTableDimensions=1  BreakpointsForDimension1=[0:1:10]  Table=10*1./(1+exp(-[0:1:10]+5))  InternalRulePriority=Speed  RndMeth=Simplest
  output current : Outport
  wires:
  Gear shifting/1 -> Scope2/1, MATLAB Function/1(Gear_Shift), If/1, Delay/1
  If/1 -> If Action Subsystem/Action
  Constant/1 -> If Action Subsystem/1(In1)
  If Action Subsystem/1(Out1) -> Sigmoid/1(In1)
  MATLAB Function/1(Output_Current) -> Scope/1, output current/1
  Sigmoid/1(Integrator) -> MATLAB Function/2(Integrator)
  Constant1/1 -> If Action Subsystem1/1(In1)
  If Action Subsystem1/1(Out1) -> Sigmoid1/1(In1)
  Delay/1 -> If/2
  If/2 -> If Action Subsystem1/Action
  Sigmoid1/1(Integrator) -> Scope1/1

== system test10/sigmoid ==
  In1 : Inport
  Constant : Constant
  Constant1 : Constant  Value=-50
  Constant2 : Constant  Value=-1
  Gain : Gain  Gain=10
  Gain1 : Gain  Gain=5
  Math Function : Math  Operator=pow
  Math Function1 : Math
  Sum : Sum  Inputs=|++
  Sum1 : Sum  Inputs=|++
  Current 1 : Outport
  wires:
  Constant1/1 -> Sum/2
  In1/1 -> Gain1/1
  Sum/1 -> Math Function1/1
  Math Function1/1 -> Sum1/2
  Constant/1 -> Sum1/1
  Constant2/1 -> Math Function/2
  Sum1/1 -> Math Function/1
  Math Function/1 -> Gain/1
  Gain/1 -> Current 1/1
  Gain1/1 -> Sum/1

== system test10/sigmoid1 ==
  In1 : Inport
  Constant : Constant
  Constant1 : Constant  Value=50
  Constant2 : Constant  Value=-1
  Gain : Gain  Gain=10
  Gain1 : Gain  Gain=-5
  Math Function : Math  Operator=pow
  Math Function1 : Math
  Sum : Sum  Inputs=|++
  Sum1 : Sum  Inputs=|++
  Current 1 : Outport
  wires:
  Constant1/1 -> Sum/2
  In1/1 -> Gain1/1
  Sum/1 -> Math Function1/1
  Math Function1/1 -> Sum1/2
  Constant/1 -> Sum1/1
  Constant2/1 -> Math Function/2
  Sum1/1 -> Math Function/1
  Math Function/1 -> Gain/1
  Gain/1 -> Current 1/1
  Gain1/1 -> Sum/1

== system test10/Clutch/RPM Sensor ==
  Mechanical Rotational Reference : fl_lib/Mechanical/Rotational Elements/Mechanical Rotational Reference
  Motion Sensor : fl_lib/Mechanical/Mechanical Sensors/Ideal Rotational Motion Sensor  reference=foundation.enum.MeasurementReference.difference  acceleration_port=false  velocity_port=true  position_port=true  wrap_angle=simscape.enum.onoff.off  offset=0 rad
  PS-Simulink Converter 2 : nesl_utility/PS-Simulink Converter  PhysicalDomain=network_engine_domain  SubClassName=ps_output  LeftPortType=input  RightPortType=output  PseudoPeriodic=off  Frequencies=[]  VectorFormat=1-D array  Unit=rpm  AffineConversion=off
  R : PMIOPort  Side=Left
  rpm : Outport  VectorParamsAs1DForOutWhenUnconnected=off
  wires:
  PS-Simulink Converter 2/1 -> rpm/1
  connections:
  R/RConn1 -- Motion Sensor/LConn1
  Motion Sensor/RConn1 -- Mechanical Rotational Reference/LConn1
  Motion Sensor/RConn2 -- PS-Simulink Converter 2/LConn1

== system test10/Clutch/RPM Sensor1 ==
  Mechanical Rotational Reference : fl_lib/Mechanical/Rotational Elements/Mechanical Rotational Reference
  Motion Sensor : fl_lib/Mechanical/Mechanical Sensors/Ideal Rotational Motion Sensor  reference=foundation.enum.MeasurementReference.difference  acceleration_port=false  velocity_port=true  position_port=true  wrap_angle=simscape.enum.onoff.off  offset=0 rad
  PS-Simulink Converter 2 : nesl_utility/PS-Simulink Converter  PhysicalDomain=network_engine_domain  SubClassName=ps_output  LeftPortType=input  RightPortType=output  PseudoPeriodic=off  Frequencies=[]  VectorFormat=1-D array  Unit=rpm  AffineConversion=off
  R : PMIOPort  Side=Left
  rpm : Outport  VectorParamsAs1DForOutWhenUnconnected=off
  wires:
  PS-Simulink Converter 2/1 -> rpm/1
  connections:
  R/RConn1 -- Motion Sensor/LConn1
  Motion Sensor/RConn1 -- Mechanical Rotational Reference/LConn1
  Motion Sensor/RConn2 -- PS-Simulink Converter 2/LConn1

== system test10/Clutch/Subsystem ==
  Input Current : Inport
  Last Output : Inport  Port=2
  Abs : Abs  SaturateOnIntegerOverflow=off
  Derivative : Derivative
  If Action Subsystem : Subsystem  TreatAsAtomicUnit=on
  If Action Subsystem1 : Subsystem  TreatAsAtomicUnit=on
  If1 : If  IfExpression=u1 <= 200
  Merge : Merge
  Scope : Scope  NumInputPorts=3
  Torque : Outport
  wires:
  Input Current/1 -> Scope/1, If Action Subsystem1/1(Input Current), Derivative/1
  If1/1 -> If Action Subsystem1/Action
  If1/2 -> If Action Subsystem/Action
  Last Output/1 -> Scope/2, If Action Subsystem/1(Last Output)
  If Action Subsystem1/1(Out1) -> Merge/1
  If Action Subsystem/1(Out1) -> Merge/2
  Merge/1 -> Scope/3, Torque/1
  Derivative/1 -> Abs/1  "I dot"
  Abs/1 -> If1/1

== system test10/Clutch/Subsystem2 ==
  Input Current : Inport
  Last Output : Inport  Port=2
  Abs : Abs  SaturateOnIntegerOverflow=off
  Derivative : Derivative
  If Action Subsystem : Subsystem  TreatAsAtomicUnit=on
  If Action Subsystem1 : Subsystem  TreatAsAtomicUnit=on
  If1 : If  IfExpression=u1 <= 200
  Merge : Merge
  Scope : Scope  NumInputPorts=3
  Torque : Outport
  wires:
  Input Current/1 -> Scope/1, If Action Subsystem1/1(Input Current), Derivative/1
  If1/1 -> If Action Subsystem1/Action
  If1/2 -> If Action Subsystem/Action
  Last Output/1 -> Scope/2, If Action Subsystem/1(Last Output)
  If Action Subsystem1/1(Out1) -> Merge/1
  If Action Subsystem/1(Out1) -> Merge/2
  Merge/1 -> Scope/3, Torque/1
  Derivative/1 -> Abs/1  "I dot"
  Abs/1 -> If1/1

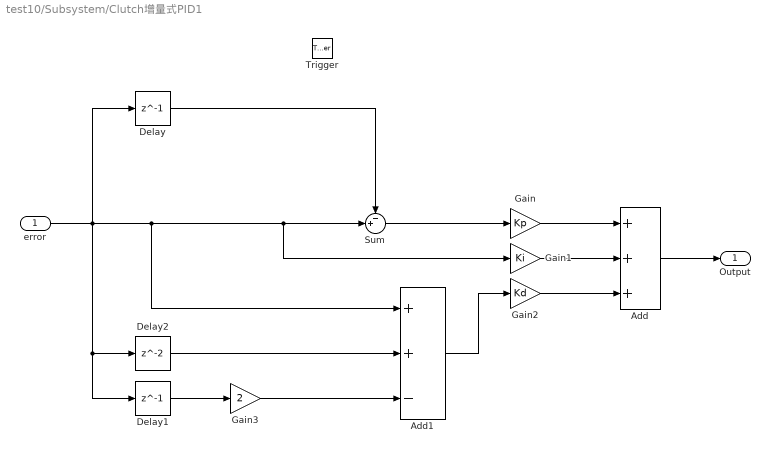
== system test10/Subsystem/Clutch增量式PID1 ==
  error : Inport
  Trigger : TriggerPort  VariantControl=(inherit)  PortDimensions=1
  Add : Sum  Inputs=+++
  Add1 : Sum  Inputs=++-
  Delay : Delay  DelayLength=1  InitialCondition=0
  Delay1 : Delay  DelayLength=1  InitialCondition=0
  Delay2 : Delay  InitialCondition=0
  Gain : Gain  Gain=Kp
  Gain1 : Gain  Gain=Ki
  Gain2 : Gain  Gain=Kd
  Gain3 : Gain  Gain=2
  Sum : Sum  Inputs=-+|
  Output : Outport
  wires:
  error/1 -> Delay1/1, Delay2/1, Add1/1, Gain1/1, Sum/2, Delay/1
  Add/1 -> Output/1
  Gain2/1 -> Add/3
  Gain1/1 -> Add/2
  Gain/1 -> Add/1
  Delay/1 -> Sum/1
  Sum/1 -> Gain/1
  Delay1/1 -> Gain3/1
  Gain3/1 -> Add1/3
  Delay2/1 -> Add1/2
  Add1/1 -> Gain2/1

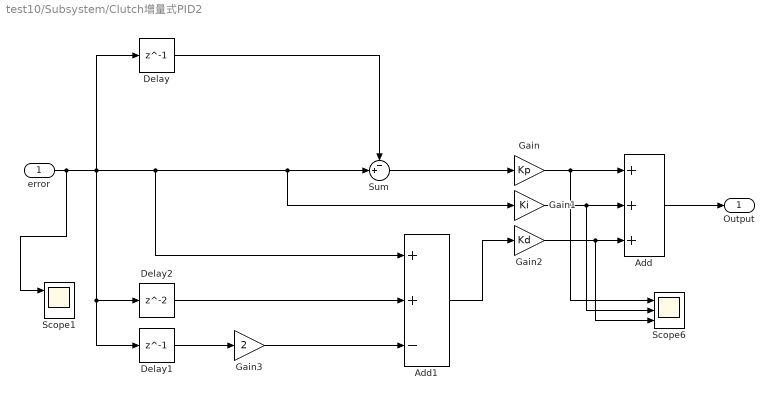
== system test10/Subsystem/Clutch增量式PID2 ==
  error : Inport
  Add : Sum  Inputs=+++
  Add1 : Sum  Inputs=++-
  Delay : Delay  DelayLength=1  InitialCondition=0
  Delay1 : Delay  DelayLength=1  InitialCondition=0
  Delay2 : Delay  InitialCondition=0
  Gain : Gain  Gain=Kp
  Gain1 : Gain  Gain=Ki
  Gain2 : Gain  Gain=Kd
  Gain3 : Gain  Gain=2
  Scope1 : Scope  NumInputPorts=3
  Scope6 : Scope  NumInputPorts=3
  Sum : Sum  Inputs=-+|
  Output : Outport
  wires:
  error/1 -> Scope1/1, Delay1/1, Delay2/1, Add1/1, Gain1/1, Sum/2, Delay/1
  Add/1 -> Output/1
  Gain2/1 -> Scope6/3, Add/3
  Gain1/1 -> Scope6/2, Add/2
  Gain/1 -> Scope6/1, Add/1
  Delay/1 -> Sum/1
  Sum/1 -> Gain/1
  Delay1/1 -> Gain3/1
  Gain3/1 -> Add1/3
  Delay2/1 -> Add1/2
  Add1/1 -> Gain2/1

== system test10/Subsystem/If Action Subsystem ==
  In1 : Inport
  Action Port : ActionPort  InitializeStates=reset  ActionPortLabel=if(u1 == 2)
  速度增量式PID1 : Subsystem  mask{Kp=2, Ki=0.1, Kd=0}
      mask DialogControl ParameterGroupVar Prompt: 参数
  Out1 : Outport
  wires:
  In1/1 -> 速度增量式PID1/1(error)
  速度增量式PID1/1(Output) -> Out1/1

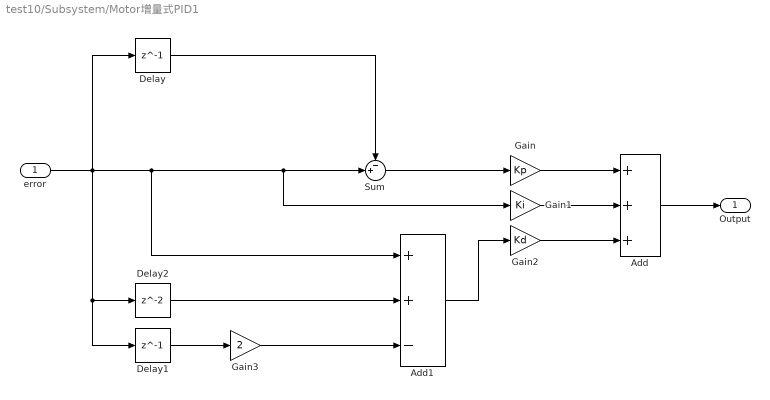
== system test10/Subsystem/Motor增量式PID1 ==
  error : Inport
  Add : Sum  Inputs=+++
  Add1 : Sum  Inputs=++-
  Delay : Delay  DelayLength=1  InitialCondition=0
  Delay1 : Delay  DelayLength=1  InitialCondition=0
  Delay2 : Delay  InitialCondition=0
  Gain : Gain  Gain=Kp
  Gain1 : Gain  Gain=Ki
  Gain2 : Gain  Gain=Kd
  Gain3 : Gain  Gain=2
  Sum : Sum  Inputs=-+|
  Output : Outport
  wires:
  error/1 -> Delay1/1, Delay2/1, Add1/1, Gain1/1, Sum/2, Delay/1
  Add/1 -> Output/1
  Gain2/1 -> Add/3
  Gain1/1 -> Add/2
  Gain/1 -> Add/1
  Delay/1 -> Sum/1
  Sum/1 -> Gain/1
  Delay1/1 -> Gain3/1
  Gain3/1 -> Add1/3
  Delay2/1 -> Add1/2
  Add1/1 -> Gain2/1

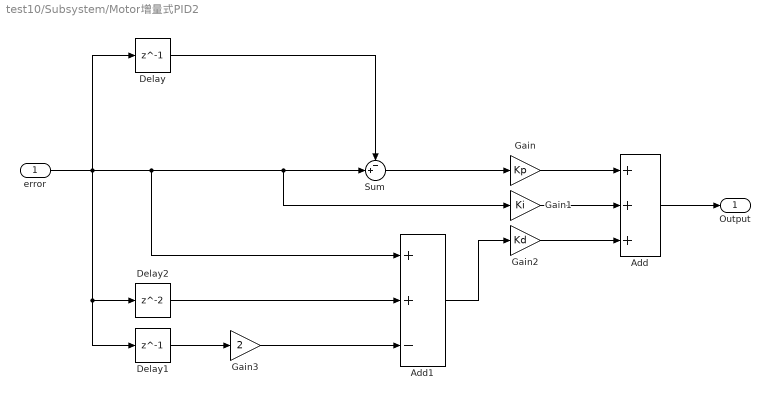
== system test10/Subsystem/Motor增量式PID2 ==
  error : Inport
  Add : Sum  Inputs=+++
  Add1 : Sum  Inputs=++-
  Delay : Delay  DelayLength=1  InitialCondition=0
  Delay1 : Delay  DelayLength=1  InitialCondition=0
  Delay2 : Delay  InitialCondition=0
  Gain : Gain  Gain=Kp
  Gain1 : Gain  Gain=Ki
  Gain2 : Gain  Gain=Kd
  Gain3 : Gain  Gain=2
  Sum : Sum  Inputs=-+|
  Output : Outport
  wires:
  error/1 -> Delay1/1, Delay2/1, Add1/1, Gain1/1, Sum/2, Delay/1
  Add/1 -> Output/1
  Gain2/1 -> Add/3
  Gain1/1 -> Add/2
  Gain/1 -> Add/1
  Delay/1 -> Sum/1
  Sum/1 -> Gain/1
  Delay1/1 -> Gain3/1
  Gain3/1 -> Add1/3
  Delay2/1 -> Add1/2
  Add1/1 -> Gain2/1

== system test10/Subsystem/Subsystem ==
  Jerk : Inport
  y : Inport  Port=2
  Enable : EnablePort
  Out1 : Outport
  Out2 : Outport  Port=2
  wires:
  Jerk/1 -> Out1/1
  y/1 -> Out2/1

== system test10/Subsystem/速度增量式PID ==
  error : Inport
  Add : Sum  Inputs=+++
  Add1 : Sum  Inputs=++-
  Delay : Delay  DelayLength=1  InitialCondition=0
  Delay1 : Delay  DelayLength=1  InitialCondition=0
  Delay2 : Delay  InitialCondition=0
  Gain : Gain  Gain=Kp
  Gain1 : Gain  Gain=Ki
  Gain2 : Gain  Gain=Kd
  Gain3 : Gain  Gain=2
  Sum : Sum  Inputs=-+|
  Output : Outport
  wires:
  error/1 -> Delay1/1, Delay2/1, Add1/1, Gain1/1, Sum/2, Delay/1
  Add/1 -> Output/1
  Gain2/1 -> Add/3
  Gain1/1 -> Add/2
  Gain/1 -> Add/1
  Delay/1 -> Sum/1
  Sum/1 -> Gain/1
  Delay1/1 -> Gain3/1
  Gain3/1 -> Add1/3
  Delay2/1 -> Add1/2
  Add1/1 -> Gain2/1

== system test10/Subsystem2/If Action Subsystem ==
  In1 : Inport
  Action Port : ActionPort  PropagateVarSize=During execution  ActionPortLabel=if(u1 == 2)
  Integrator : Integrator
  Out1 : Outport
  wires:
  In1/1 -> Integrator/1
  Integrator/1 -> Out1/1

== system test10/Subsystem2/If Action Subsystem1 ==
  In1 : Inport
  Action Port : ActionPort  InitializeStates=reset  PropagateVarSize=During execution  ActionPortLabel=elseif(u1 == 1)
  Integrator : Integrator
  Out1 : Outport
  wires:
  In1/1 -> Integrator/1
  Integrator/1 -> Out1/1

== system test10/Subsystem2/Sigmoid ==
  In1 : Inport
  Constant1 : Constant
  Constant2 : Constant  Value=-8
  Constant3 : Constant  Value=-1
  Gain : Gain  Gain=10
  Gain1 : Gain  Gain=100
  Math Function : Math  Operator=pow
  Math Function1 : Math
  Scope : Scope  NumInputPorts=2
  Sum : Sum  Inputs=|++
  Sum1 : Sum  Inputs=|++
  Integrator : Outport
  wires:
  Constant1/1 -> Sum1/1
  Sum1/1 -> Math Function/1
  Constant3/1 -> Math Function/2
  Sum/1 -> Math Function1/1
  Math Function/1 -> Gain/1
  Gain1/1 -> Sum/1
  Gain/1 -> Integrator/1, Scope/1
  Math Function1/1 -> Sum1/2
  Constant2/1 -> Sum/2
  In1/1 -> Gain1/1

== system test10/Subsystem2/Sigmoid1 ==
  In1 : Inport
  Constant1 : Constant
  Constant2 : Constant  Value=8
  Constant3 : Constant  Value=-1
  Gain : Gain  Gain=10
  Gain1 : Gain  Gain=-100
  Math Function : Math  Operator=pow
  Math Function1 : Math
  Scope : Scope  NumInputPorts=2
  Sum : Sum  Inputs=|++
  Sum1 : Sum  Inputs=|++
  Integrator : Outport
  wires:
  Constant1/1 -> Sum1/1
  Sum1/1 -> Math Function/1
  Constant3/1 -> Math Function/2
  Sum/1 -> Math Function1/1
  Math Function/1 -> Gain/1
  Gain1/1 -> Sum/1
  Gain/1 -> Integrator/1, Scope/1
  Math Function1/1 -> Sum1/2
  Constant2/1 -> Sum/2
  In1/1 -> Gain1/1

== system test10/Clutch/Subsystem/If Action Subsystem ==
  Last Output : Inport
  Action Port : ActionPort  PropagateVarSize=During execution  ActionPortLabel=else
  Out1 : Outport
  wires:
  Last Output/1 -> Out1/1

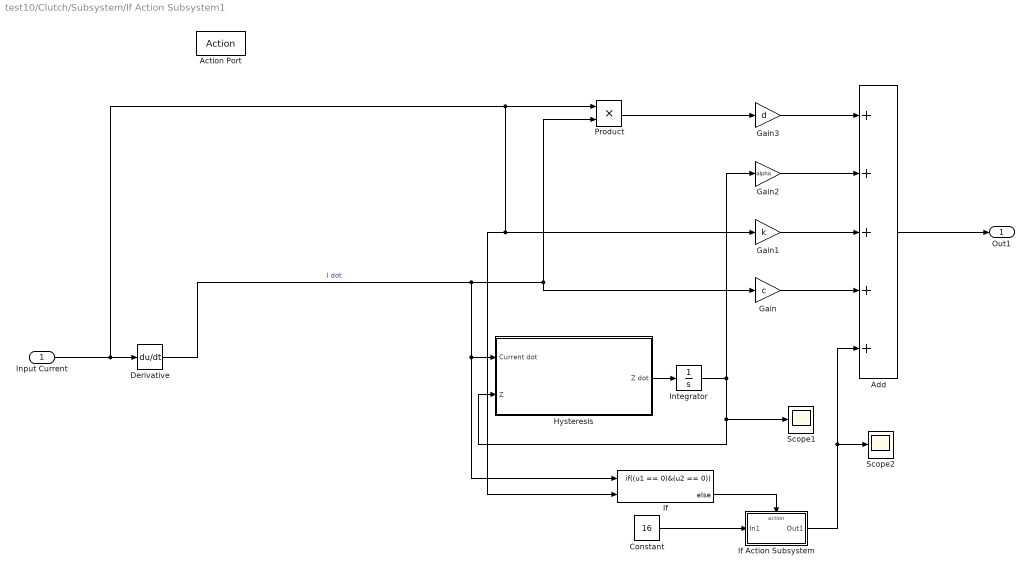
== system test10/Clutch/Subsystem/If Action Subsystem1 ==
  Input Current : Inport
  Action Port : ActionPort  InitializeStates=reset  PropagateVarSize=During execution  ActionPortLabel=if(u1 <= 200)
  Add : Sum  Inputs=+++++
  Constant : Constant  Value=16
  Derivative : Derivative
  Gain : Gain  Gain=c
  Gain1 : Gain  Gain=k
  Gain2 : Gain  Gain=alpha
  Gain3 : Gain  Gain=d
  Hysteresis : Subsystem  mask{theta=-0.41731, beta=-0.83796, v=2.2221, gamma=2.0211}
  If : If  NumInputs=2  IfExpression=(u1 == 0)&(u2 == 0)
  If Action Subsystem : Subsystem  TreatAsAtomicUnit=on
  Integrator : Integrator
  Product : Product
  Scope1 : Scope
  Scope2 : Scope
  Out1 : Outport
  wires:
  Gain1/1 -> Add/3
  Gain/1 -> Add/4
  Derivative/1 -> If/1, Hysteresis/1(Current dot), Product/2, Gain/1  "I dot"
  Product/1 -> Gain3/1
  Constant/1 -> If Action Subsystem/1(In1)
  If/2 -> If Action Subsystem/Action
  Add/1 -> Out1/1
  Hysteresis/1(Z dot) -> Integrator/1
  Input Current/1 -> If/2, Gain1/1, Product/1, Derivative/1
  Integrator/1 -> Scope1/1, Hysteresis/2(Z), Gain2/1
  Gain3/1 -> Add/1
  Gain2/1 -> Add/2
  If Action Subsystem/1(Out1) -> Scope2/1, Add/5

== system test10/Clutch/Subsystem2/If Action Subsystem ==
  Last Output : Inport
  Action Port : ActionPort  PropagateVarSize=During execution  ActionPortLabel=else
  Out1 : Outport
  wires:
  Last Output/1 -> Out1/1

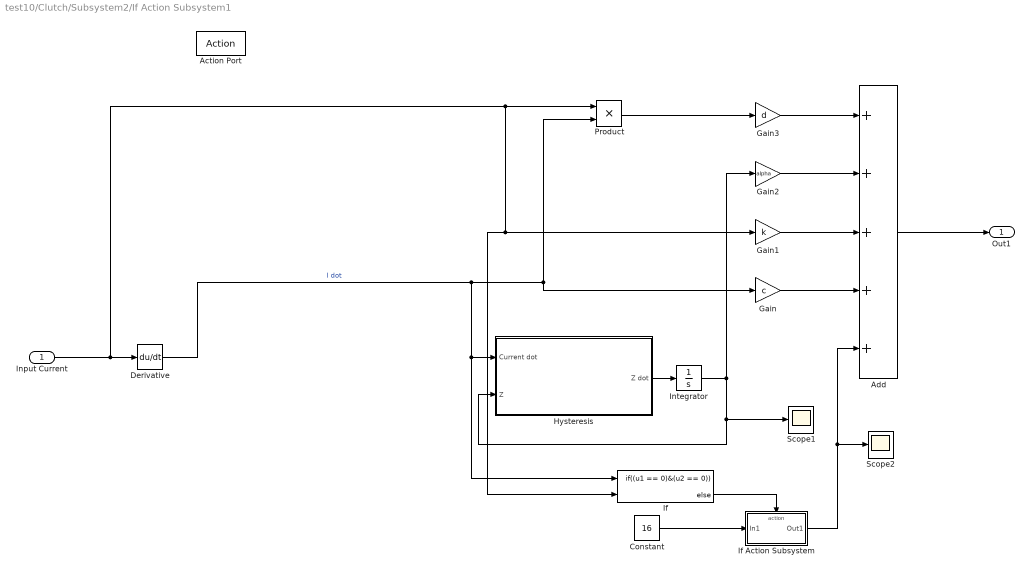
== system test10/Clutch/Subsystem2/If Action Subsystem1 ==
  Input Current : Inport
  Action Port : ActionPort  InitializeStates=reset  PropagateVarSize=During execution  ActionPortLabel=if(u1 <= 200)
  Add : Sum  Inputs=+++++
  Constant : Constant  Value=16
  Derivative : Derivative
  Gain : Gain  Gain=c
  Gain1 : Gain  Gain=k
  Gain2 : Gain  Gain=alpha
  Gain3 : Gain  Gain=d
  Hysteresis : Subsystem  mask{theta=-0.41731, beta=-0.83796, v=2.2221, gamma=2.0211}
  If : If  NumInputs=2  IfExpression=(u1 == 0)&(u2 == 0)
  If Action Subsystem : Subsystem  TreatAsAtomicUnit=on
  Integrator : Integrator
  Product : Product
  Scope1 : Scope
  Scope2 : Scope
  Out1 : Outport
  wires:
  Gain1/1 -> Add/3
  Gain/1 -> Add/4
  Derivative/1 -> If/1, Hysteresis/1(Current dot), Product/2, Gain/1  "I dot"
  Product/1 -> Gain3/1
  Constant/1 -> If Action Subsystem/1(In1)
  If/2 -> If Action Subsystem/Action
  Add/1 -> Out1/1
  Hysteresis/1(Z dot) -> Integrator/1
  Input Current/1 -> If/2, Gain1/1, Product/1, Derivative/1
  Integrator/1 -> Scope1/1, Hysteresis/2(Z), Gain2/1
  Gain3/1 -> Add/1
  Gain2/1 -> Add/2
  If Action Subsystem/1(Out1) -> Scope2/1, Add/5

== system test10/Subsystem/If Action Subsystem/速度增量式PID1 ==
  error : Inport
  Add : Sum  Inputs=+++
  Add1 : Sum  Inputs=++-
  Delay : Delay  DelayLength=1  InitialCondition=0
  Delay1 : Delay  DelayLength=1  InitialCondition=0
  Delay2 : Delay  InitialCondition=0
  Gain : Gain  Gain=Kp
  Gain1 : Gain  Gain=Ki
  Gain2 : Gain  Gain=Kd
  Gain3 : Gain  Gain=2
  Sum : Sum  Inputs=-+|
  Output : Outport
  wires:
  error/1 -> Delay1/1, Delay2/1, Add1/1, Gain1/1, Sum/2, Delay/1
  Add/1 -> Output/1
  Gain2/1 -> Add/3
  Gain1/1 -> Add/2
  Gain/1 -> Add/1
  Delay/1 -> Sum/1
  Sum/1 -> Gain/1
  Delay1/1 -> Gain3/1
  Gain3/1 -> Add1/3
  Delay2/1 -> Add1/2
  Add1/1 -> Gain2/1

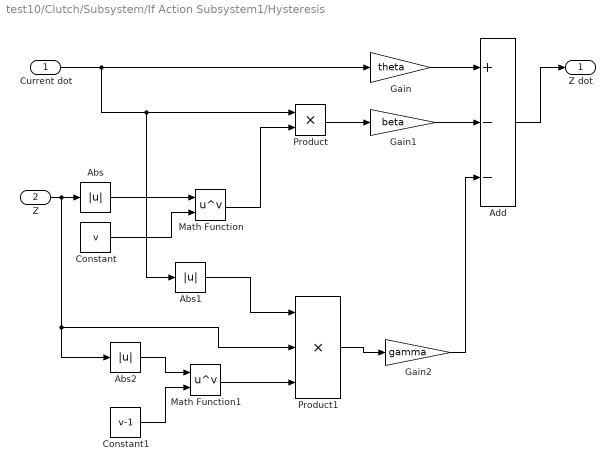
== system test10/Clutch/Subsystem/If Action Subsystem1/Hysteresis ==
  Current dot : Inport
  Z : Inport  Port=2
  Abs : Abs  SaturateOnIntegerOverflow=off
  Abs1 : Abs  SaturateOnIntegerOverflow=off
  Abs2 : Abs  SaturateOnIntegerOverflow=off
  Add : Sum  Inputs=+--
  Constant : Constant  Value=v
  Constant1 : Constant  Value=v-1
  Gain : Gain  Gain=theta
  Gain1 : Gain  Gain=beta
  Gain2 : Gain  Gain=gamma
  Math Function : Math  Operator=pow
  Math Function1 : Math  Operator=pow
  Product : Product
  Product1 : Product  Inputs=3
  Z dot : Outport
  wires:
  Current dot/1 -> Abs1/1, Product/1, Gain/1
  Gain/1 -> Add/1
  Z/1 -> Product1/2, Abs2/1, Abs/1
  Math Function/1 -> Product/2
  Product/1 -> Gain1/1
  Gain1/1 -> Add/2
  Math Function1/1 -> Product1/3
  Abs1/1 -> Product1/1
  Add/1 -> Z dot/1
  Abs/1 -> Math Function/1
  Constant/1 -> Math Function/2
  Product1/1 -> Gain2/1
  Gain2/1 -> Add/3
  Abs2/1 -> Math Function1/1
  Constant1/1 -> Math Function1/2

== system test10/Clutch/Subsystem/If Action Subsystem1/If Action Subsystem ==
  In1 : Inport
  Action Port : ActionPort  ActionPortLabel=else
  Out1 : Outport
  wires:
  In1/1 -> Out1/1

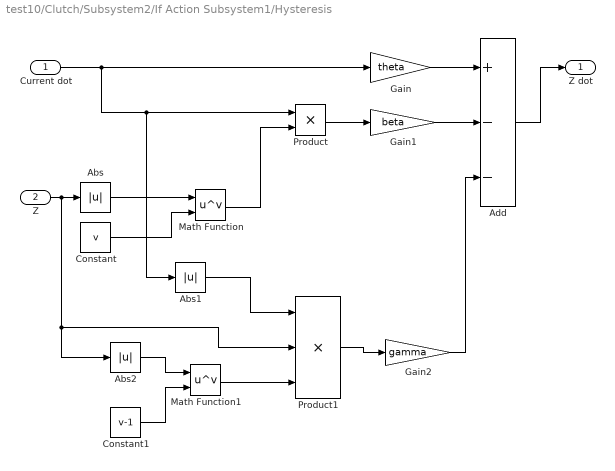
== system test10/Clutch/Subsystem2/If Action Subsystem1/Hysteresis ==
  Current dot : Inport
  Z : Inport  Port=2
  Abs : Abs  SaturateOnIntegerOverflow=off
  Abs1 : Abs  SaturateOnIntegerOverflow=off
  Abs2 : Abs  SaturateOnIntegerOverflow=off
  Add : Sum  Inputs=+--
  Constant : Constant  Value=v
  Constant1 : Constant  Value=v-1
  Gain : Gain  Gain=theta
  Gain1 : Gain  Gain=beta
  Gain2 : Gain  Gain=gamma
  Math Function : Math  Operator=pow
  Math Function1 : Math  Operator=pow
  Product : Product
  Product1 : Product  Inputs=3
  Z dot : Outport
  wires:
  Current dot/1 -> Abs1/1, Product/1, Gain/1
  Gain/1 -> Add/1
  Z/1 -> Product1/2, Abs2/1, Abs/1
  Math Function/1 -> Product/2
  Product/1 -> Gain1/1
  Gain1/1 -> Add/2
  Math Function1/1 -> Product1/3
  Abs1/1 -> Product1/1
  Add/1 -> Z dot/1
  Abs/1 -> Math Function/1
  Constant/1 -> Math Function/2
  Product1/1 -> Gain2/1
  Gain2/1 -> Add/3
  Abs2/1 -> Math Function1/1
  Constant1/1 -> Math Function1/2

== system test10/Clutch/Subsystem2/If Action Subsystem1/If Action Subsystem ==
  In1 : Inport
  Action Port : ActionPort  ActionPortLabel=else
  Out1 : Outport
  wires:
  In1/1 -> Out1/1

== matlab function test10/Subsystem/MATLAB Function2 ==
  data: u input; y output
function y = fcn(u)

if u < 0
    y = 0;
elseif u> 10
    y = 10;
else
    y = u;
end

== matlab function test10/Clutch/MATLAB Function1 ==
  data: boundary input; output_torque output; input_torque input
function output_torque = fcn(boundary, input_torque)

if (boundary <= 0) || (input_torque <= 0)
    output_torque = 0;
else
    if input_torque < boundary
        output_torque = input_torque;
    else
        output_torque = boundary;
    end
end

== matlab function test10/Clutch/MATLAB Function2 ==
  data: boundary input; output_torque output; input_torque input
function output_torque = fcn(boundary, input_torque)

if (boundary <= 0) || (input_torque <= 0)
    output_torque = 0;
else
    if input_torque < boundary
        output_torque = input_torque;
    else
        output_torque = boundary;
    end
end

== matlab function test10/Clutch/MATLAB Function ==
  data: Gear_1 input; Gear_Shifting output; Gear_2 input; Speed input
function Gear_Shifting = fcn(Gear_1, Gear_2, Speed)

if (Gear_2 > 4500)||(Speed > 60)
    Gear_Shifting = 2;
else
    Gear_Shifting = 1;
end

== matlab function test10/Subsystem2/MATLAB Function ==
  data: Gear_Shift input; Integrator input; Output_Current output
function Output_Current  = fcn(Gear_Shift, Integrator)

if Gear_Shift == 1
    Output_Current = 10;
else
    Output_Current = Integrator;
end

== matlab function test10/Subsystem/MATLAB Function1 ==
  data: u input; y output; Dead_Area input
function y = fcn(u,Dead_Area)

if (abs(u) >= Dead_Area) && (u< 0)
    y = -1*u ; 
elseif (abs(u) >= Dead_Area) && (u > 0)
       y = -1*u; 
else
 y = 0;
end
